simulink model "ds_simple_twovav"  (R2020a)
settings: Solver=ode1be  StartTime=0.0  StopTime=24*3600  FixedStep=0.001  RelTol=1e-3
PostLoadFcn:
  | if any(exist('dsrtsu_mdlpostloadfcn', 'file') ~= 0), dsrtsu_mdlpostloadfcn('Execute', bdroot); end
InitFcn:
  | , if any(exist('rtifpga_mdlclblib', 'file') ~= 0), rtifpga_mdlclblib('Init', bdroot); end,
  | , if any(exist('dsmpb_private', 'file') ~= 0), dsmpb_private('dsmpb_mdlclblib', 'Init', bdroot); end,
libraries: neural x4, dsmpblib x4
PreSaveFcn:
  | , if any(exist('dsmpb_private', 'file') ~= 0), dsmpb_private('dsmpb_mdlclblib', 'PreSave', bdroot); end,
CloseFcn:
  | , if any(exist('dsmpb_private', 'file') ~= 0), dsmpb_private('dsmpb_mdlclblib', 'Close', bdroot); end,
settings Model: RTICANMMDATA=struct('GeneralSetupData',struct('modelroot','D:\github\dspace-modelica-example\dSpaceExample','generalsettings',struct('filesettings',struct('destfolder',struct('Name','RTICANMM_FILES','Check',1),'buildfolder',struct('Name','.','Check',1),'AbsDestfolder',struct('Name','D:\github\dspace-modelica-example\dSpaceExample\RTICANMM_FILES'),'AbsBuildfolder',struct('Name','D:\github\dspace-modelica-example\dSpaceExample'))),'options',struct('addpaths',1,'rmpaths',1,'addtrcexclusion',true,'cannavigator',struct('checkmonitoring',0),'show_usrtrc',0,'use_usrtrc',0),'advanced',struct('options',ones(1,100)),'MPSetup',{{}},'RTI',struct('Type','DSRT','Ver','4.3','Date','02-May-2020'),'modelname','ds_simple_twovav','block','ds_simple_twovav'))  DSRTSU_INTERNAL_RTIFPGA=160  DSMPB_ID_DATA={'236',struct('BlockId','db60070b-df7b-44ed-b750-cfd2b2fb3f9f','SignalIds',{{'bb3a5f76-9421-4e74-869d-1121775f016d'}}),'237',struct('BlockId','e9b9945a-31f3-4010-a8f7-35b42b310d19','SignalIds',{{'9f4600a4-f050-4de3-b65c-a4e916c07273'}}),'238',struct('BlockId','2c11abef-c5d0-4944-bc68-9310ebf6e01f','SignalIds',{{'04ba7a63-2602-44d5-947f-4ac2f5006d2b'}}),'239',struct('BlockId','d057b1e2-fe3b-4b69-9a22-ac3e68195dda','SignalIds',{{'77330597-c16e-4df2-9510-155471efb7bd'}}),'240',struct('BlockId','08f95fd0-40cf-47d5-ab4c-59a75cfa282c','SignalIds',{{'eadba8ad-2dab-4e97-8c0a-c4e323ad4b42'}}),'241',struct('BlockId','b5e1c2c7-b317-4633-bd12-793f49455b19','SignalIds',{{'9e9eef31-2180-474d-8328-a0ce75ef502c'}}),'242',struct('BlockId','be52a969-daf4-4d41-81e7-d2965b038824','SignalIds',{{'88cc5638-5a4d-4050-80e5-e1a520294fcc'}})}  Creator=yangyang.fu  LastModifiedBy=yangyang.fu
settings OptimizationCC: BlockReduction=off  ConditionallyExecuteInputs=off  OptimizeBlockIOStorage=off  BufferReuse=off
settings DebuggingCC: TasksWithSamePriorityMsg=none
settings HardwareCC: ProdBitPerPointer=32  ProdBitPerSizeT=32  ProdBitPerPtrDiffT=32  ProdLargestAtomicInteger=Integer  ProdWordSize=32  ProdLongLongMode=on  ProdHWDeviceType=Custom Processor->Custom
settings ModelReferenceCC: EnableParallelModelReferenceBuilds=on
settings SFSimCC: MATLABDynamicMemAlloc=off
settings RTWCC: Description=dSPACE Run-Time Target (for VEOS on Windows and ConfigurationDesk)  SystemTargetFile=dsrt.tlc  GenCodeOnly=on  MakeCommand=make_dsrt  TemplateMakefile=dsrt_default_tmf  RTWVerbose=off  CustomInclude="\"C:\\Program Files\\Dymola 2021\\Source\" \"D:\\github\\dspace-modelica-example\\Libraries\\Buildings 7.0.0\\Resources\\C-Sources\""
settings STFCustomTargetCC: TargetLangStandard=C99 (ISO)  ParMdlRefBuildCompliant=on  SystemTargetFile=dsrt.tlc
settings GRTTargetCC: CompOptLevelCompliant=off  ConcurrentExecutionCompliant=off  CombineOutputUpdateFcns=off  MatFileLogging=off  CPPClassGenCompliant=off  UseToolchainInfoCompliant=off

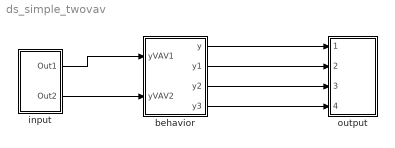
== system ds_simple_twovav ==
  behavior : Subsystem
  input : Subsystem
  output : Subsystem
  wires:
  input/1(Out1) -> behavior/1(yVAV1)
  input/2(Out2) -> behavior/2(yVAV2)
  behavior/1(y) -> output/1(Voltage)
  behavior/2(y1) -> output/2(Voltage1)
  behavior/3(y2) -> output/3(Voltage2)
  behavior/4(y3) -> output/4(Voltage3)

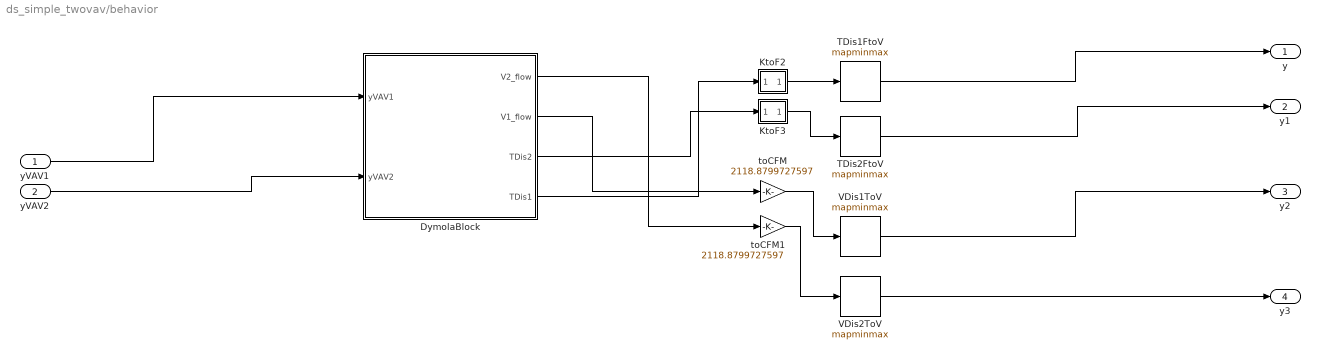
== system ds_simple_twovav/behavior ==
  yVAV1 : Inport
  yVAV2 : Inport  Port=2
  DymolaBlock : Subsystem  Tag=20-Oct-2021 18:01:18#5469
      mask help:
      | Dymola block.
      | A dymola block allows acausal physical modeling.
      | See Dymola manual for usage.
      settings: CopyFcn=newDymolaGui('20-Oct-2021 18:01:18#5469','Copy');  DeleteFcn=if exist('newDymolaGui') newDymolaGui('ds_simple_twovav/behavior/DymolaBlock','Delete'); end;  NameChangeFcn=newDymolaGui('20-Oct-2021 18:01:18#5469','Copy');  OpenFcn=newDymolaGui('ds_simple_twovav/behavior/DymolaBlock','Init');
      mask Display: image(reshape([1;1;1;1;1;1;1;1;1;1;1;1;1;1;1;1;1;1;1;1;1;1;0;0;0;0;0;0;0;0;0;0;1;1;1;1;1;1;1;1;0;1;1;1;1;1;1;1;1;0;1;1;1;1;1;0;0;0;0;0;0;0;1;1;0;0;0;0;0;0;0;1;1;0;0;0;0;0;0;0;1;1;0;0;0;0;0;0;0;1;1;0;0;0;0;0;0;0;1;1;0;0;0;0;0;0;0;1;1;0;0;0;0;0;0;0;1;1;0;0;0;0;0;0;0;1;1;0;0;0;0;0;0;0;1;1;0;0;0;0;0;0;0;1;1;0;0;0;0;0;0;0;1;1;0;0;0;0;0;0;0;1;1;0;0;0;0;0;0;0;1;1;0;0;0;0;0;0;0;1;1;0;0;0;0;0;0;0;1;1;0;0;0;0;0;0;0;1;1;0;0;0;0;0;0;0;1;1;0;0;0;0;0;0;0;1;1;0;0;0;0;0;0;0;1;1;0;0;0;0;0;0;0;1;1;0;0;0;0;0;0;0;1;1;0;0;0;0;0;0;0;1;1;0;0;0;0;0;0;0;1;1;0;0;0;0;0;0;0;1;1;1;1;1;0;1;1;1;1;1;1;1;1;0;1;1;1;1;1;1;1;1;0;0;0;0;0;0;0;0;0;0;1;1;1;1;1;1;1;1;1;1;1;1;1;1;1;1;1;1;1;1;1;1;1;1;1;1;1;1;1;1;1;1;1;1;1;1;1;1;1;1;1;1;1;1;0;0;0;0;0;0;0;0;0;0;1;1;1;1;1;1;1;1;0;1;1;1;1;1;1;1;1;0;1;1;1;1;1;0;0;0;0;0;0;0;1;1;0;0;0;0;0;0;0;1;1;0;0;0;0;0;0;0;1;1;0;0;0;0;0;0;0;1;1;0;0;0;0;0;0;0;1;1;0;0;0;0;0;0;0;1;1;0;0;0;0;0;0;0;1;1;0;0;0;0;0;0;0;1;1;0;0;0;0;0;0;0;1;1;0;0;0;0;0;0;0;1;1;0;0;0;0;0;0;0;1;1;0;0;0;0;0;0;0;1;1;0;0;0;0;0;0;0;1;1;0;0;0;0;0;0;0;1;1;0;0;0;0;0;0;0;1;1;0;0;0;0;0;0;0;1;1;0;0;0;0;0;0;0;1;1;0;0;0;0;0;0;0;1;1;0;0;0;0;0;0;0;1;1;0;0;0;0;0;0;0;1;1;0;0;0;0;0;0;0;1;1;0;0;0;0;0;0;0;1;1;0;0;0;0;0;0;0;1;1;0;0;0;0;0;0;0;1;1;1;1;1;0;1;1;1;1;1;1;1;1;0;1;1;1;1;1;1;1;1;0;0;0;0;0;0;0;0;0;0;1;1;1;1;1;1;1;1;1;1;1;1;1;1;1;1;1;1;1;1;1;1;1;1;1;1;1;1;1;1;1;1;1;1;1;1;1;1;1;1;1;1;1;1;0;0;0;0;0;0;0;0;0;0;1;1;1;1;1;1;1;1;0;1;1;1;1;1;1;1;1;0;1;1;1;1;1;0;0;0;0;0;0;0;1;1;0;0;0;0;0;0;0;1;1;0;1;1;1;1;1;0;1;1;0;1;1;1;1;1;0;1;1;0;1;1;1;1;1;0;1;1;0;1;1;1;1;1;0;1;1;0;1;1;1;1;1;0;1;1;0;1;1;1;1;1;0;1;1;0;1;1;1;1;1;0;1;1;0;1;1;1;1;1;0;1;1;0;1;1;1;1;1;0;1;1;0;1;1;1;1;1;0;1;1;0;1;1;1;1;1;0;1;1;0;1;1;1;1;1;0;1;1;0;1;1;1;1;1;0;1;1;0;1;1;1;1;1;0;1;1;0;1;1;1;1;1;0;1;1;0;1;1;1;1;1;0;1;1;0;1;1;1;1;1;0;1;1;0;1;1;1;1;1;0;1;1;0;1;1;1;1;1;0;1;1;0;1;1;1;1;1;0;1;1;0;0;0;0;0;0;0;1;1;0;0;0;0;0;0;0;1;1;1;1;1;0;1;1;1;1;1;1;1;1;0;1;1;1;1;1;1;1;1;0;0;0;0;0;0;0;0;0;0;1;1;1;1;1;1;1;1;1;1;1;1;1;1;1;1;1;1;1;1;1;1],18,18,3),[.2,.2,.6,.6])
  KtoF2 : Subsystem
  KtoF3 : Subsystem
  TDis1FtoV : neural/Processing Functions/mapminmax  xmin=-150  xmax=150  ymin=-10  ymax=+10
  TDis2FtoV : neural/Processing Functions/mapminmax  xmin=-150  xmax=150  ymin=-10  ymax=+10
  VDis1ToV : neural/Processing Functions/mapminmax  xmin=0  xmax=20000  ymin=-10  ymax=+10
  VDis2ToV : neural/Processing Functions/mapminmax  xmin=0  xmax=20000  ymin=-10  ymax=+10
  toCFM : Gain  Gain=2118.8799727597
  toCFM1 : Gain  Gain=2118.8799727597
  y : Outport
  y1 : Outport  Port=2
  y2 : Outport  Port=3
  y3 : Outport  Port=4
  wires:
  TDis2FtoV/1 -> y1/1
  KtoF3/1(Out1) -> TDis2FtoV/1
  toCFM/1 -> VDis1ToV/1
  DymolaBlock/3(TDis2) -> KtoF3/1(In1)
  VDis2ToV/1 -> y3/1
  DymolaBlock/2(V1_flow) -> toCFM/1
  KtoF2/1(Out1) -> TDis1FtoV/1
  DymolaBlock/4(TDis1) -> KtoF2/1(In1)
  DymolaBlock/1(V2_flow) -> toCFM1/1
  toCFM1/1 -> VDis2ToV/1
  TDis1FtoV/1 -> y/1
  VDis1ToV/1 -> y2/1
  yVAV2/1 -> DymolaBlock/2(yVAV2)
  yVAV1/1 -> DymolaBlock/1(yVAV1)

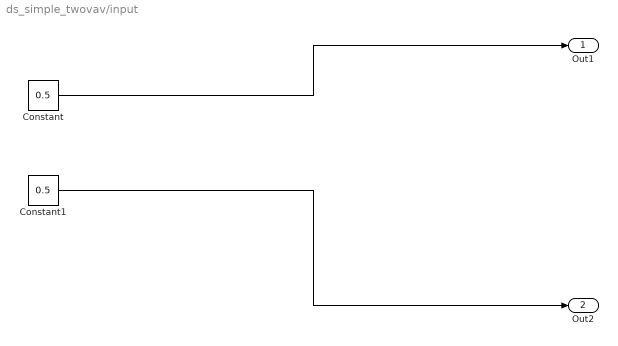
== system ds_simple_twovav/input ==
  Constant : Constant  Value=0.5  SampleTime=0.01
  Constant1 : Constant  Value=0.5  SampleTime=0.01
  Out1 : Outport
  Out2 : Outport  Port=2
  wires:
  Constant/1 -> Out1/1
  Constant1/1 -> Out2/1

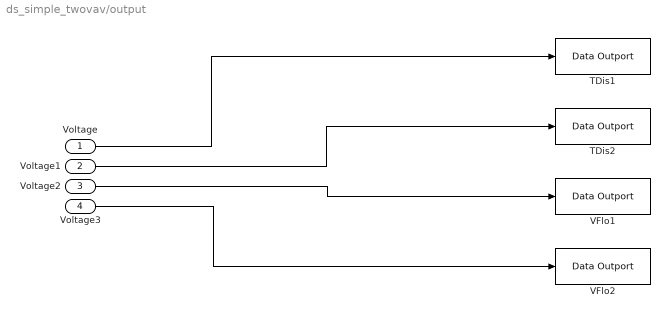
== system ds_simple_twovav/output ==
  Voltage : Inport
  Voltage1 : Inport  Port=2
  Voltage2 : Inport  Port=3
  Voltage3 : Inport  Port=4
  TDis1 : dsmpblib/Data Outport  Priority=-10000
      settings: SourceProductName=dSPACE Model Interface Blockset
  TDis2 : dsmpblib/Data Outport  Priority=-10000
      settings: SourceProductName=dSPACE Model Interface Blockset
  VFlo1 : dsmpblib/Data Outport  Priority=-10000
      settings: SourceProductName=dSPACE Model Interface Blockset
  VFlo2 : dsmpblib/Data Outport  Priority=-10000
      settings: SourceProductName=dSPACE Model Interface Blockset
  wires:
  Voltage2/1 -> VFlo1/1
  Voltage/1 -> TDis1/1
  Voltage1/1 -> TDis2/1
  Voltage3/1 -> VFlo2/1

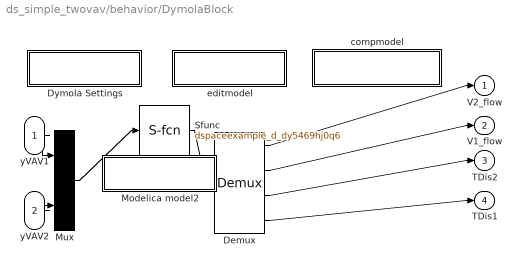
== system ds_simple_twovav/behavior/DymolaBlock ==
  yVAV1 : Inport
  yVAV2 : Inport  Port=2
  Demux : Demux  Outputs=[1;1;1;1]
  Dymola Settings : Subsystem  mask{ModelName=dSpaceExample.Debug.TwoVAVTerminals, MoFileName=D:/github/dspace-modelica-example/dSpaceExample/Debug/TwoVAVTerminals.mo, dSpace=, BusConnector=[], ResultFile=[], ResultFileOnline=[], ResultDt=[], Libs=:, bigobj=[], ImportFolder=[], guimode=[], ModelName2=[], forRuntime=[], MEXLoad=[], omitDescription=[], ResultName=dspaceexample_d_dy5469hj0q6}
      mask prompts: ModelName "Name of Dymola model"; MoFileName "File Name (including .mo)"; ResultFile "Create Result"; ResultFileOnline "Load result"; ResultDt "Result min dt"; Libs "Used Libraries"; bigobj "Compiler flag /bigobj"; ImportFolder "Import folder"; guimode "GUI mode flag"; ModelName2 "Model name for import mode"; forRuntime "Runtime export"; MEXLoad "Compiled S-function"; omitDescription "Omit description strings"; ResultName "Name of result file"
      mask Display: disp('Dymola Settings');
  Modelica model2 : Subsystem
      mask Display: disp('Change parameters');
  Mux : Mux  Inputs=[1;1]
  Sfunc : S-Function  Tag=5469hj0q6  FunctionName=dspaceexample_d_dy5469hj0q6  Parameters=[VRoo;vav1_vav_sta_default_p;vav1_vav_sta_default_T;vav1_vav_sta_default_X;vav1_vav_riseTime;vav1_vav_y_start;vav1_vav_filter_gain;vav1_vav_filter_A_ripple;vav1_vav_filter_f_min;vav1_vav_filter_normalize10;vav1_vav_filter_x_start;vav1_vav_filter_u_nominal;vav1_vav_use_deltaM;vav1_vav_deltaM;vav1_vav_roundDuct;vav1_vav_ReC;vav1_vav_a;vav1_vav_b;vav1_vav_yL;vav1_vav_yU;vav1_vav_k1;vav1_vav_l;vav1_vav_l2;vav1_vav_deltax;vav1_vav_y_min;vav1_terHea_bal1_preDro_s26;vav1_terHea_bal1_preDro_s27;vav1_terHea_bal1_preDro_s28;vav1_terHea_bal2_preDro_s29;vav1_terHea_bal2_preDro_s30;vav1_terHea_delta;vav1_terHea_T_a1_nominal;vav1_terHea_T_a2_nominal;vav1_terHea_r_nominal;vav1_terHea_hA_n_w;vav1_terHea_hA_n_a;vav1_terHea_hA_T0_w;vav1_terHea_hA_T0_a;vav1_sinTer_X;vav1_sinTer_p;vav1_sinTer_T;vav1_souTer_X;vav1_souTer_m_flow;vav1_souTer_T;zer_k;rooSin_p;rooSin_T;rooSin_X;vav2_vav_sta_default_p;vav2_vav_sta_default_T;vav2_vav_sta_default_X;vav2_vav_riseTime;vav2_vav_y_start;vav2_vav_filter_gain;vav2_vav_filter_A_ripple;vav2_vav_filter_f_min;vav2_vav_filter_normalize57;vav2_vav_filter_x_start;vav2_vav_filter_u_nominal;vav2_vav_use_deltaM;vav2_vav_deltaM;vav2_vav_roundDuct;vav2_vav_ReC;vav2_vav_a;vav2_vav_b;vav2_vav_yL;vav2_vav_yU;vav2_vav_k1;vav2_vav_l;vav2_vav_l2;vav2_vav_deltax;vav2_vav_y_min;vav2_terHea_bal1_preDro_s73;vav2_terHea_bal1_preDro_s74;vav2_terHea_bal1_preDro_s75;vav2_terHea_bal2_preDro_s76;vav2_terHea_bal2_preDro_s77;vav2_terHea_delta;vav2_terHea_T_a1_nominal;vav2_terHea_T_a2_nominal;vav2_terHea_r_nominal;vav2_terHea_hA_n_w;vav2_terHea_hA_n_a;vav2_terHea_hA_T0_w;vav2_terHea_hA_T0_a;vav2_sinTer_X;vav2_sinTer_p;vav2_sinTer_T;vav2_souTer_X;vav2_souTer_m_flow;vav2_souTer_T;coiSou_X;coiSou_T;byp_sta_default_p;byp_sta_default_T;byp_sta_default_X;VSup2_T_start;VSup2_p_start;VSup2_X_start;VSup1_T_start;VSup1_p_start;VSup1_X_start;TDisVAV1_T_start;TDisVAV1_TAmb;TDisVAV1_tauHeaTra;TDisVAV2_T_start;TDisVAV2_TAmb;TDisVAV2_tauHeaTra],[]  PortCounts=[1;1]  SFunctionDeploymentMode=off  EnableBusSupport=off  mask{VRoo=129.6, vav1_vav_sta_default_p=101325, vav1_vav_sta_default_T=293.15, vav1_vav_sta_default_X=[0.01; 0.99], vav1_vav_riseTime=120, vav1_vav_y_start=1, vav1_vav_filter_gain=1, vav1_vav_filter_A_ripple=0.5, vav1_vav_filter_f_min=0, vav1_vav_filter_normalize10=1, vav1_vav_filter_x_start=[0; 0], vav1_vav_filter_u_nominal=1, vav1_vav_use_deltaM=1, vav1_vav_deltaM=0.3, vav1_vav_roundDuct=0, vav1_vav_ReC=4000, vav1_vav_a=-1.51, vav1_vav_b=9.45, vav1_vav_yL=0.166666666666667, vav1_vav_yU=0.611111111111111, vav1_vav_k1=0.45, vav1_vav_l=0.0001, vav1_vav_l2=0.01, vav1_vav_deltax=0.02, vav1_vav_y_min=0.02, vav1_terHea_bal1_preDro_s26=101325, vav1_terHea_bal1_preDro_s27=293.15, vav1_terHea_bal1_preDro_s28=[0.01; 0.99], vav1_terHea_bal2_preDro_s29=300000, vav1_terHea_bal2_preDro_s30=293.15, vav1_terHea_delta=0.001, vav1_terHea_T_a1_nominal=289.85, vav1_terHea_T_a2_nominal=355.35, vav1_terHea_r_nominal=0.666666666666667, vav1_terHea_hA_n_w=0.85, vav1_terHea_hA_n_a=0.8, vav1_terHea_hA_T0_w=293.15, vav1_terHea_hA_T0_a=293.15, vav1_sinTer_X=1, vav1_sinTer_p=300000, vav1_sinTer_T=293.15, vav1_souTer_X=1, vav1_souTer_m_flow=0, vav1_souTer_T=323.15, zer_k=0, rooSin_p=101325, rooSin_T=293.15, rooSin_X=[0.01; 0.99], vav2_vav_sta_default_p=101325, vav2_vav_sta_default_T=293.15, vav2_vav_sta_default_X=[0.01; 0.99], vav2_vav_riseTime=120, vav2_vav_y_start=1, vav2_vav_filter_gain=1, vav2_vav_filter_A_ripple=0.5, vav2_vav_filter_f_min=0, vav2_vav_filter_normalize57=1, vav2_vav_filter_x_start=[0; 0], vav2_vav_filter_u_nominal=1, vav2_vav_use_deltaM=1, vav2_vav_deltaM=0.3, vav2_vav_roundDuct=0, vav2_vav_ReC=4000, vav2_vav_a=-1.51, vav2_vav_b=9.45, vav2_vav_yL=0.166666666666667, vav2_vav_yU=0.611111111111111, vav2_vav_k1=0.45, vav2_vav_l=0.0001, vav2_vav_l2=0.01, vav2_vav_deltax=0.02, vav2_vav_y_min=0.02, vav2_terHea_bal1_preDro_s73=101325, vav2_terHea_bal1_preDro_s74=293.15, vav2_terHea_bal1_preDro_s75=[0.01; 0.99], vav2_terHea_bal2_preDro_s76=300000, vav2_terHea_bal2_preDro_s77=293.15, vav2_terHea_delta=0.001, vav2_terHea_T_a1_nominal=289.85, vav2_terHea_T_a2_nominal=355.35, vav2_terHea_r_nominal=0.666666666666667, vav2_terHea_hA_n_w=0.85, vav2_terHea_hA_n_a=0.8, vav2_terHea_hA_T0_w=293.15, vav2_terHea_hA_T0_a=293.15, vav2_sinTer_X=1, vav2_sinTer_p=300000, vav2_sinTer_T=293.15, vav2_souTer_X=1, vav2_souTer_m_flow=0, vav2_souTer_T=323.15, coiSou_X=[0.01; 0.99], coiSou_T=285.15, byp_sta_default_p=101325, byp_sta_default_T=293.15, byp_sta_default_X=[0.01; 0.99], VSup2_T_start=293.15, VSup2_p_start=101325, VSup2_X_start=[0.01; 0.99], VSup1_T_start=293.15, VSup1_p_start=101325, VSup1_X_start=[0.01; 0.99], TDisVAV1_T_start=293.15, TDisVAV1_TAmb=293.15, TDisVAV1_tauHeaTra=1200, TDisVAV2_T_start=293.15, TDisVAV2_TAmb=293.15, TDisVAV2_tauHeaTra=1200}
      mask prompts: vav1_vav_sta_default_p "vav1.vav.sta_default.p"; vav1_vav_sta_default_T "vav1.vav.sta_default.T"; vav1_vav_sta_default_X "vav1.vav.sta_default.X"; vav1_vav_riseTime "vav1.vav.riseTime"; vav1_vav_y_start "vav1.vav.y_start"; vav1_vav_filter_gain "vav1.vav.filter.gain"; vav1_vav_filter_A_ripple "vav1.vav.filter.A_ripple"; vav1_vav_filter_f_min "vav1.vav.filter.f_min"; vav1_vav_filter_normalize10 "vav1.vav.filter.normalized"; vav1_vav_filter_x_start "vav1.vav.filter.x_start"; vav1_vav_filter_u_nominal "vav1.vav.filter.u_nominal"; vav1_vav_use_deltaM "vav1.vav.use_deltaM"; vav1_vav_deltaM "vav1.vav.deltaM"; vav1_vav_roundDuct "vav1.vav.roundDuct"; vav1_vav_ReC "vav1.vav.ReC"; vav1_vav_a "vav1.vav.a"; vav1_vav_b "vav1.vav.b"; vav1_vav_yL "vav1.vav.yL"; vav1_vav_yU "vav1.vav.yU"; vav1_vav_k1 "vav1.vav.k1"; vav1_vav_l "vav1.vav.l"; vav1_vav_l2 "vav1.vav.l2"; vav1_vav_deltax "vav1.vav.deltax"; vav1_vav_y_min "vav1.vav.y_min"; vav1_terHea_bal1_preDro_s26 "vav1.terHea.bal1.preDro.sta_default.p"; vav1_terHea_bal1_preDro_s27 "vav1.terHea.bal1.preDro.sta_default.T"; vav1_terHea_bal1_preDro_s28 "vav1.terHea.bal1.preDro.sta_default.X"; vav1_terHea_bal2_preDro_s29 "vav1.terHea.bal2.preDro.sta_default.p"; vav1_terHea_bal2_preDro_s30 "vav1.terHea.bal2.preDro.sta_default.T"; vav1_terHea_delta "vav1.terHea.delta"; vav1_terHea_T_a1_nominal "vav1.terHea.T_a1_nominal"; vav1_terHea_T_a2_nominal "vav1.terHea.T_a2_nominal"; vav1_terHea_r_nominal "vav1.terHea.r_nominal"; vav1_terHea_hA_n_w "vav1.terHea.hA.n_w"; vav1_terHea_hA_n_a "vav1.terHea.hA.n_a"; vav1_terHea_hA_T0_w "vav1.terHea.hA.T0_w"; vav1_terHea_hA_T0_a "vav1.terHea.hA.T0_a"; vav1_sinTer_X "vav1.sinTer.X"; vav1_sinTer_p "vav1.sinTer.p"; vav1_sinTer_T "vav1.sinTer.T"; vav1_souTer_X "vav1.souTer.X"; vav1_souTer_m_flow "vav1.souTer.m_flow"; vav1_souTer_T "vav1.souTer.T"; zer_k "zer.k"; rooSin_p "rooSin.p"; rooSin_T "rooSin.T"; rooSin_X "rooSin.X"; vav2_vav_sta_default_p "vav2.vav.sta_default.p"; vav2_vav_sta_default_T "vav2.vav.sta_default.T"; vav2_vav_sta_default_X "vav2.vav.sta_default.X"; vav2_vav_riseTime "vav2.vav.riseTime"; vav2_vav_y_start "vav2.vav.y_start"; vav2_vav_filter_gain "vav2.vav.filter.gain"; vav2_vav_filter_A_ripple "vav2.vav.filter.A_ripple"; vav2_vav_filter_f_min "vav2.vav.filter.f_min"; vav2_vav_filter_normalize57 "vav2.vav.filter.normalized"; vav2_vav_filter_x_start "vav2.vav.filter.x_start"; vav2_vav_filter_u_nominal "vav2.vav.filter.u_nominal"; vav2_vav_use_deltaM "vav2.vav.use_deltaM"; vav2_vav_deltaM "vav2.vav.deltaM"; vav2_vav_roundDuct "vav2.vav.roundDuct"; vav2_vav_ReC "vav2.vav.ReC"; vav2_vav_a "vav2.vav.a"; vav2_vav_b "vav2.vav.b"; vav2_vav_yL "vav2.vav.yL"; vav2_vav_yU "vav2.vav.yU"; vav2_vav_k1 "vav2.vav.k1"; vav2_vav_l "vav2.vav.l"; vav2_vav_l2 "vav2.vav.l2"; vav2_vav_deltax "vav2.vav.deltax"; vav2_vav_y_min "vav2.vav.y_min"; vav2_terHea_bal1_preDro_s73 "vav2.terHea.bal1.preDro.sta_default.p"; vav2_terHea_bal1_preDro_s74 "vav2.terHea.bal1.preDro.sta_default.T"; vav2_terHea_bal1_preDro_s75 "vav2.terHea.bal1.preDro.sta_default.X"; vav2_terHea_bal2_preDro_s76 "vav2.terHea.bal2.preDro.sta_default.p"; vav2_terHea_bal2_preDro_s77 "vav2.terHea.bal2.preDro.sta_default.T"; vav2_terHea_delta "vav2.terHea.delta"; vav2_terHea_T_a1_nominal "vav2.terHea.T_a1_nominal"; vav2_terHea_T_a2_nominal "vav2.terHea.T_a2_nominal"; vav2_terHea_r_nominal "vav2.terHea.r_nominal"; vav2_terHea_hA_n_w "vav2.terHea.hA.n_w"; vav2_terHea_hA_n_a "vav2.terHea.hA.n_a"; vav2_terHea_hA_T0_w "vav2.terHea.hA.T0_w"; vav2_terHea_hA_T0_a "vav2.terHea.hA.T0_a"; vav2_sinTer_X "vav2.sinTer.X"; vav2_sinTer_p "vav2.sinTer.p"; vav2_sinTer_T "vav2.sinTer.T"; vav2_souTer_X "vav2.souTer.X"; vav2_souTer_m_flow "vav2.souTer.m_flow"; vav2_souTer_T "vav2.souTer.T"; coiSou_X "coiSou.X"; coiSou_T "coiSou.T"; byp_sta_default_p "byp.sta_default.p"; byp_sta_default_T "byp.sta_default.T"; byp_sta_default_X "byp.sta_default.X"; VSup2_T_start "VSup2.T_start"; VSup2_p_start "VSup2.p_start"; VSup2_X_start "VSup2.X_start"; VSup1_T_start "VSup1.T_start"; VSup1_p_start "VSup1.p_start"; VSup1_X_start "VSup1.X_start"; TDisVAV1_T_start "TDisVAV1.T_start"; TDisVAV1_TAmb "TDisVAV1.TAmb"; TDisVAV1_tauHeaTra "TDisVAV1.tauHeaTra"; TDisVAV2_T_start "TDisVAV2.T_start"; TDisVAV2_TAmb "TDisVAV2.TAmb"; TDisVAV2_tauHeaTra "TDisVAV2.tauHeaTra"
      mask Display: image(imread('Dymola.bmp'))
  compmodel : Subsystem
      settings: OpenFcn=compileModelica('ds_simple_twovav/behavior/DymolaBlock');
      mask Display: disp('Compile Modelica model');
  editmodel : Subsystem
      settings: OpenFcn=editModelica('ds_simple_twovav/behavior/DymolaBlock');
      mask Display: disp('Edit Modelica model');
  V2_flow : Outport
  V1_flow : Outport  Port=2
  TDis2 : Outport  Port=3
  TDis1 : Outport  Port=4
  wires:
  Sfunc/1 -> Demux/1
  Demux/1 -> V2_flow/1
  Demux/2 -> V1_flow/1
  Demux/3 -> TDis2/1
  Demux/4 -> TDis1/1
  Mux/1 -> Sfunc/1
  yVAV1/1 -> Mux/1
  yVAV2/1 -> Mux/2

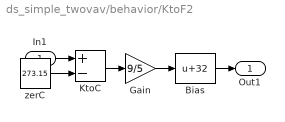
== system ds_simple_twovav/behavior/KtoF2 ==
  In1 : Inport
  Bias : Bias  Bias=32
  Gain : Gain  Gain=9/5
  KtoC : Sum  Inputs=+-
  zerC : Constant  Value=273.15  SampleTime=0
  Out1 : Outport
  wires:
  Gain/1 -> Bias/1
  KtoC/1 -> Gain/1
  zerC/1 -> KtoC/2
  Bias/1 -> Out1/1
  In1/1 -> KtoC/1

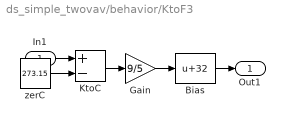
== system ds_simple_twovav/behavior/KtoF3 ==
  In1 : Inport
  Bias : Bias  Bias=32
  Gain : Gain  Gain=9/5
  KtoC : Sum  Inputs=+-
  zerC : Constant  Value=273.15  SampleTime=0
  Out1 : Outport
  wires:
  Gain/1 -> Bias/1
  KtoC/1 -> Gain/1
  zerC/1 -> KtoC/2
  Bias/1 -> Out1/1
  In1/1 -> KtoC/1

== system ds_simple_twovav/behavior/DymolaBlock/Dymola Settings ==

== system ds_simple_twovav/behavior/DymolaBlock/Modelica model2 ==

== system ds_simple_twovav/behavior/DymolaBlock/compmodel ==

== system ds_simple_twovav/behavior/DymolaBlock/editmodel ==
